simulink model "random_model"  (Simulink 8.4)
settings: Solver=ode45  StartTime=0.0  StopTime=inf  RelTol=1e-3
settings Model: Creator=2110973l  LastModifiedBy=2110973l
settings DataIOCC: SignalLoggingSaveFormat=Dataset
settings OptimizationCC: ExpressionDepthLimit=128
settings DebuggingCC: UnderspecifiedInitializationDetection=Simplified  MergeDetectMultiDrivingBlocksExec=error  FcnCallInpInsideContextMsg=EnableAllAsError  StateNameClashWarn=none
settings GRTTargetCC: CombineOutputUpdateFcns=on  GRTInterface=off

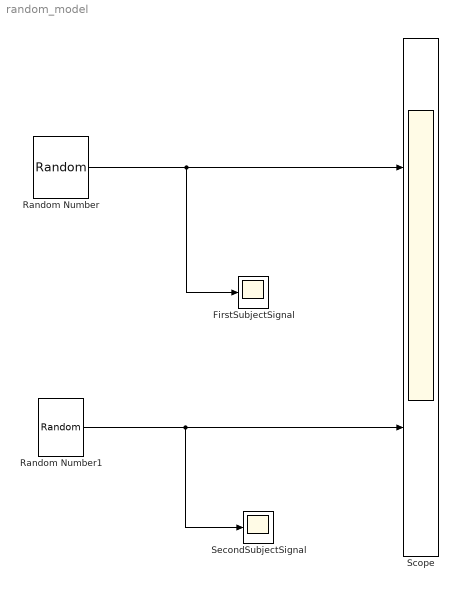
== system random_model ==
  FirstSubjectSignal : Scope
  Random Number : RandomNumber  Mean=2  SampleTime=0.5
  Random Number1 : RandomNumber  Mean=1  Variance=2  SampleTime=0.5
  Scope : Scope  NumInputPorts=2
      settings: YMin=-0.5~-2  YMax=4.5~5
  SecondSubjectSignal : Scope
      settings: SaveName=ScopeData2
  wires:
  Random Number/1 -> FirstSubjectSignal/1, Scope/1
  Random Number1/1 -> SecondSubjectSignal/1, Scope/2
